simulink model "Vehicle_Model_Controller_may29_mod"  (R2020b)
settings: Solver=VariableStepAuto  StartTime=0.0  StopTime=15  FixedStep=0.015  MaxStep=0.1  RelTol=1e-3
model workspace (MAT data in the model file):
  Kp = 10
  understeer_gradient = 0.05
values from neighbouring files (symbols this model uses):
  inch2mm = 25.4    [e_diff.m]
  S1 = 7 * (10^(-5))    (= 7e-05)    [e_diff.m]
  S2 = -0.0038    [e_diff.m]
  S3 = 0.6535    [e_diff.m]
  S4 = 0.1061    [e_diff.m]
  steer_slope = 0.00962    [e_diff.m]
undefined symbols (not defined in the file or in its folder): DiscIntNeverNeededParam
libraries: fl_lib x24, nesl_utility x22, sdl_lib x6, autolibshared x1, autolibdatasheetbattery x1
(part 2 of 2)

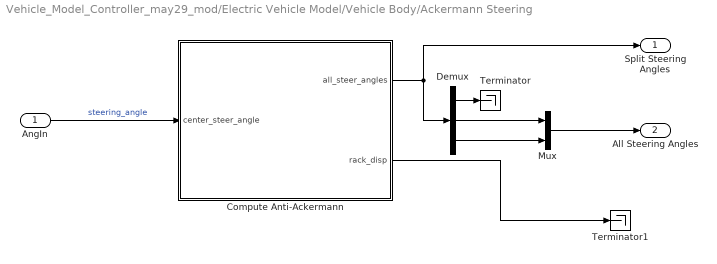
== system Vehicle_Model_Controller_may29_mod/Electric Vehicle Model/Vehicle Body/Ackermann Steering ==
  AngIn : Inport
  Compute Anti-Ackermann : MATLAB Function  TreatAsAtomicUnit=on
  Demux : Demux  Outputs=3
  Mux : Mux  Inputs=2
  Terminator : Terminator
  Terminator1 : Terminator
  Split Steering Angles : Outport
  All Steering Angles : Outport  Port=2
  wires:
  Demux/1 -> Terminator/1
  Compute Anti-Ackermann/1(all_steer_angles) -> Demux/1, Split Steering Angles/1
  Demux/3 -> Mux/2
  AngIn/1 -> Compute Anti-Ackermann/1(center_steer_angle)  "steering_angle"
  Demux/2 -> Mux/1
  Mux/1 -> All Steering Angles/1
  Compute Anti-Ackermann/2(rack_disp) -> Terminator1/1

== matlab function Vehicle_Model_Controller_may29_mod/RWD Control/MATLAB Function1 ==
  data: omega_m output; AP input; t_req output; Vx input; yaw input; sensor_left_wheel_speed output; sensor_right_wheel_speed output
function [omega_m, t_req, sensor_left_wheel_speed, sensor_right_wheel_speed] = pre_process(AP, Vx, yaw)
%% Constants
r = 0.22; % Tire radius [m]
GR_r = (40/21) * (84/23) + 1; % Rear gear ratio [Unitless]
gr = [GR_r, GR_r]; % Gear ratios [Unitless]
max_torque = 4095;
s = [0.647895, 0.62102]; % Half track width [front rear][m]

sensor_left_wheel_speed = Vx + (yaw * s(2));
sensor_right_wheel_speed = Vx + (yaw * -s(2));

Vx_tires = [sensor_left_wheel_speed sensor_right_wheel_speed];
omega_m = Vx_tires .* (gr ./ r);

t_req = int16(max_torque .* AP);
end

== matlab function Vehicle_Model_Controller_may29_mod/RWD Control/MATLAB Function ==
  data: AP input; Vx input; Tx output size=[1 2]; sensor_left_wheel_speed input; sensor_right_wheel_speed input; sensor_steering_wheel_angle input; yaw input; filter_yaw input; prev_Tx input; filter_yaw output
function [Tx, filter_yaw]  = e_diff_c(AP, Vx, sensor_left_wheel_speed, sensor_right_wheel_speed, sensor_steering_wheel_angle, yaw, filter_yaw, prev_Tx)
% force single instead of MATLAB default double
torque_output_left = int16(0);
torque_output_right = int16(0);
filter_yaw_s = single(filter_yaw);

TxL = int16(prev_Tx(1));
TxR = int16(prev_Tx(2));

coder.cinclude("eDiff.h");

% use pass by address to output Tx
coder.ceval("eDiff", AP, sensor_left_wheel_speed, sensor_right_wheel_speed, Vx, ...
    sensor_steering_wheel_angle, TxL, TxR, yaw, coder.ref(filter_yaw_s), coder.ref(torque_output_left), coder.ref(torque_output_right));

Tx = double([torque_output_left, torque_output_right]);
filter_yaw = double(filter_yaw_s);

end

== matlab function Vehicle_Model_Controller_may29_mod/Electric Vehicle Model/Vehicle Body/Ackermann Steering/Compute Anti-Ackermann ==
  data: center_steer_angle input; all_steer_angles output size=[1 3]; S1 parameter; S2 parameter; S3 parameter; S4 parameter; inch2mm parameter; steer_slope parameter; deg2rad parameter; rack_disp output
function [all_steer_angles, rack_disp]  = anti_ackermann(center_steer_angle, S1, S2, S3, S4, inch2mm, steer_slope, deg2rad)
rack_disp = steer_slope * inch2mm * center_steer_angle;

left_steer_angle = -((S1*(-rack_disp)^3)+(S2*(-rack_disp)^2)+(S3*-rack_disp)+S4);
right_steer_angle = ((S1*(rack_disp)^3)+(S2*(rack_disp)^2)+(S3*rack_disp)+S4);

all_steer_angles = [center_steer_angle left_steer_angle right_steer_angle].*deg2rad;

end

== matlab function Vehicle_Model_Controller_may29_mod/Motor and Battery/Motors/  ==
  data: ang_vel_RPM input; motor_torque output size=[1 2]; torque_request input
function motor_torque = get_torque(ang_vel_RPM, torque_request)
%% Actual Torque Output
% Developers:    Demetrius Gulewicz

% Developed for: Purdue Electric Racing
% Date:          09/18/2021
%
% Definitions:
% ang_vel:   Angular velocity of each wheel on the wheel fixed y axis [RPM]
% torque_request: Requested torque from the LP model                  [Nm]

%% Constants
% quadratic constants that connect current and max RPM of motors
a_v = 0.2667;
b_v = -66.353;
c_v = 10452 - ang_vel_RPM;

% quadratic constants that connnect current and max torque of motors
a_t = -0.0987;
b_t = 45.799;
c_t = -129.65;

% maximum possible current at the current RPM
max_current = [0, 0];


%% Calculate Maximum Torque Possible
% calculate the maximum current possible at the current RPM
for i = [1:2]
   if ang_vel_RPM(i) < 7000
       max_current(i) = 70;
   else
       max_current(i) = (-b_v - sqrt(b_v^2 - (4*a_v.*c_v(i)))) .* (1/(2*a_v));
   end
end

% calculate the meximum torque at the max current
max_torque = (a_t .* (max_current.^2)) + (b_t .* max_current) + c_t;
for i = [1:2]
   if max_torque(i) < 0
      max_torque(i) = 0;
   end
end

motor_torque_matrix = [max_torque; torque_request'];
motor_torque = min(motor_torque_matrix);

== matlab function Vehicle_Model_Controller_may29_mod/Electric Vehicle Model/Vehicle Body/MATLAB Function ==
  data: Vy input; Vx input; Fext output
function Fext = get_downforce(Vy, Vx)
%% Constants
rho = 1.225; % Air density [Kg/m^3]
cl = 2.11014; % Lift coefficient [unitless]
A = 1.0221; % Frontal Area [m^2]


%% Computation
% Compute CoG Velocity
Vcog = Vx^2 + Vy^2;

% Compute DownForce
Fz = 0.5 * rho * Vcog * cl * A;
Fext = [0, 0, Fz];

== matlab function Vehicle_Model_Controller_may29_mod/Electric Vehicle Model/MATLAB Function ==
  data: FwF output; FX input; FwR output
function [FwF, FwR] = fcn(FX)
%% Construct Force Matrix
FwF = FX(1:2);
FwR = FX(3:4);

== matlab function Vehicle_Model_Controller_may29_mod/RWD Control/MATLAB Function2 ==
  data: Vx input; SA output; Vy input; yaw input; center_steer_angle input
function SA = fcn(Vx, Vy, yaw, center_steer_angle)
steer_slope = 0.00962; % [in/deg] 
inch2mm = 25.4; % [mm/in]
deg2rad = 0.01745329; % [rad/deg]

S1 = 7 * (10^(-5));
S2 = -0.0038;
S3 = 0.6535;
S4 = 0.1061;


rack_disp = steer_slope * inch2mm * center_steer_angle;

left_steer_angle = -((S1*(-rack_disp)^3)+(S2*(-rack_disp)^2)+(S3*-rack_disp)+S4);
right_steer_angle = ((S1*(rack_disp)^3)+(S2*(rack_disp)^2)+(S3*rack_disp)+S4);

all_steer_angles = [center_steer_angle left_steer_angle right_steer_angle].*deg2rad;


Vg = [Vx, Vy];
s = [0.647895, 0.62102]; % Half track width [front rear][m]
l = [0.7922471, 0.7828529]; % Wheelbase [front rear][m]


% Individual slip angles, it blows up at low velocity
if abs(Vg(1)) > 0.1
    phi_fl = atan2(Vy + (l(1)*yaw), Vx + (s(1)*yaw));
    phi_fr = atan2(Vy + (l(1)*yaw), Vx - (s(1)*yaw));
    phi_rl = atan2(Vy - (l(2)*yaw), Vx + (s(2)*yaw));
    phi_rr = atan2(Vy - (l(2)*yaw), Vx - (s(2)*yaw));
else
    phi_fl = 0;
    phi_fr = 0;
    phi_rl = 0;
    phi_rr = 0;
end

phi = [phi_fl phi_fr phi_rl phi_rr];

% Compute Slip Angle
SA_fl = -phi_fl + (left_steer_angle * deg2rad);
SA_fr = -phi_fr + (right_steer_angle * deg2rad);
SA_rl = -phi_rl;
SA_rr = -phi_rr;

SA = [SA_fl SA_fr SA_rl SA_rr] ./ deg2rad;

== matlab function Vehicle_Model_Controller_may29_mod/Motor and Battery/Motors/   ==
  data: Battery_Voltage input; ang_vel_RAD input; battery_current output; Motor_torque input; battery_power output
function [battery_current, battery_power]= get_batt_curr(Battery_Voltage, ang_vel_RAD, Motor_torque)
%% Current Draw
% Developers:    Demetrius Gulewicz

% Developed for: Purdue Electric Racing
% Date:          09/18/2021
%
% Definitions:
% ang_vel_RAD:   Angular velocity of each wheel on the wheel fixed y axis [RAD]
% Motor_torque:  Torque the motor actually outputs                 [Ncm]
% Battery_Voltage: The voltage of the battery                      [V]

%% Definitions
a = 0.0411;
b = 2.7976;
c = 45.978;

t = Motor_torque;
w = ang_vel_RAD;
v = Battery_Voltage;

e = 85;

%% Calculate Current Draw
%x0 = [20, 20, 20, 20];
%options = optimoptions('fsolve','Algorithm','Levenberg-Marquardt');
%F = @(x) ([(a * x(1)^3) + (b * x(1)^2) + (c * x(1)), ] .* v) - (t .* w);
%battery_current = sum(fsolve(F,x0,options));
% 
% battery_current = sum((t .* w') ./ (e .* v));
% battery_power = battery_current * Battery_Voltage;

battery_current = [0 0];
battery_power = [0 0];

end
